simulink model "expertSystem"  (R2020a)
settings: Solver=ode45  StartTime=0.0  StopTime=0.25  FixedStep=1e-2  MaxStep=1e-2  RelTol=1e-3  EnableMultiTasking=on
StartFcn:
  | close all
StopFcn:
  | myStop()
libraries: simulink x15
settings Model: SimulationMode=accelerator  Creator=marcelo  LastModifiedBy=debora
settings SolverCC: ZeroCrossAlgorithm=Non-adaptive  AlgebraicLoopSolver=LineSearch
settings DataIOCC: SaveFormat=Array  SignalLoggingSaveFormat=ModelDataLogs  SaveOutput=off  ReturnWorkspaceOutputs=off
settings OptimizationCC: ExpressionDepthLimit=2147483647  InitFltsAndDblsToZero=on  LifeSpan=inf
settings DebuggingCC: SaveWithParameterizedLinksMsg=none  UnderspecifiedInitializationDetection=Classic  MergeDetectMultiDrivingBlocksExec=none  SignalResolutionControl=TryResolveAllWithWarning  SolverPrmCheckMsg=warning  MultiTaskDSMMsg=warning  MultiTaskCondExecSysMsg=none  FcnCallInpInsideContextMsg=warning  StateNameClashWarn=warning  SFUnexpectedBacktrackingDiag=warning  SFNoUnconditionalDefaultTransitionDiag=warning  SFExecutionAtInitializationDiag=none  ArithmeticOperatorsInVariantConditions=warning
settings HardwareCC: ProdBitPerPointer=32  ProdBitPerSizeT=32  ProdBitPerPtrDiffT=32  ProdLargestAtomicFloat=None  ProdIntDivRoundTo=Undefined  ProdEndianess=Unspecified  ProdWordSize=32  ProdHWDeviceType=32-bit Generic
settings ModelReferenceCC: PropagateSignalLabelsOutOfModel=off
settings CodeAppCC: StateflowObjectComments=on
settings GRTTargetCC: TargetFcnLib=ansi_tfl_tmw.mat  TargetLangStandard=C89/C90 (ANSI)  CombineOutputUpdateFcns=off  GRTInterface=on
settings ConfigComp: CovMetricSettings=dw  CovHtmlReporting=on  CovSaveCumulativeToWorkspaceVar=on  CovSaveSingleToWorkspaceVar=on

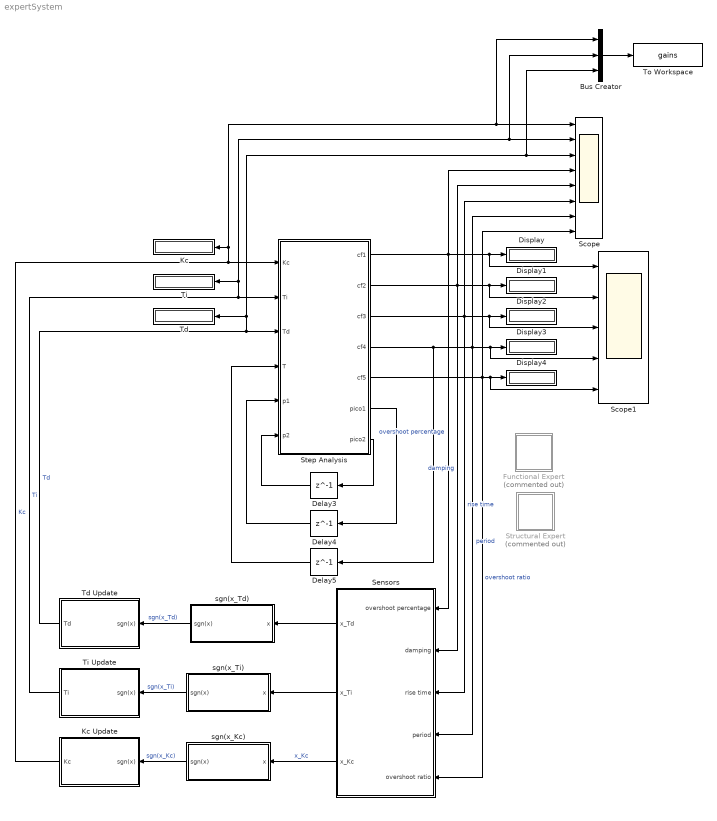
== system expertSystem ==
  Bus Creator : BusCreator  Inputs=3
  Delay3 : Delay  DelayLength=1
  Delay4 : Delay  DelayLength=1
  Delay5 : Delay  DelayLength=1
  Display{,1..4} (5 alike) : Display
  Functional Expert : Subsystem  Commented=on
  Kc : Display
  Kc Update : Subsystem
  Scope : Scope  NumInputPorts=8
  Scope1 : Scope  NumInputPorts=5
  Sensors : Subsystem
  Step Analysis : MATLAB Function  TreatAsAtomicUnit=on
  Structural Expert : Subsystem  Commented=on
  Td : Display
  Td Update : Subsystem
  Ti : Display
  Ti Update : Subsystem
  To Workspace : ToWorkspace  VariableName=gains  SampleTime=-1
      settings: Save2DSignal=2-D array (concatenate along first dimension)
  sgn(x_Kc) : Subsystem
  sgn(x_Td) : Subsystem
  sgn(x_Ti) : Subsystem
  wires:
  Step Analysis/1(cf1) -> Scope/4, Scope1/1, Display/1, Sensors/1(overshoot percentage)  "overshoot percentage"
  Step Analysis/2(cf2) -> Sensors/2(damping), Scope/5, Scope1/2, Display1/1  "damping"
  Step Analysis/3(cf3) -> Scope1/3, Display2/1, Sensors/3(rise time), Scope/6  "rise time"
  Step Analysis/4(cf4) -> Delay5/1, Sensors/4(period), Scope/7, Scope1/4, Display3/1  "period"
  Step Analysis/5(cf5) -> Sensors/5(overshoot ratio), Scope/8, Scope1/5, Display4/1  "overshoot ratio"
  Step Analysis/7(pico2) -> Delay3/1
  Step Analysis/6(pico1) -> Delay4/1
  Delay3/1 -> Step Analysis/6(p2)
  Delay4/1 -> Step Analysis/5(p1)
  Delay5/1 -> Step Analysis/4(T)
  Td Update/1(Td) -> Step Analysis/3(Td), Bus Creator/3, Scope/3, Td/1  "Td"
  Sensors/3(x_Kc) -> sgn(x_Kc)/1(x)  "x_Kc"
  sgn(x_Kc)/1(sgn(x)) -> Kc Update/1(sgn(x))  "sgn(x_Kc)"
  Kc Update/1(Kc) -> Bus Creator/1, Scope/1, Kc/1, Step Analysis/1(Kc)  "Kc"
  Sensors/2(x_Ti) -> sgn(x_Ti)/1(x)
  Sensors/1(x_Td) -> sgn(x_Td)/1(x)
  sgn(x_Td)/1(sgn(x)) -> Td Update/1(sgn(x))  "sgn(x_Td)"
  sgn(x_Ti)/1(sgn(x)) -> Ti Update/1(sgn(x))  "sgn(x_Ti)"
  Ti Update/1(Ti) -> Step Analysis/2(Ti), Bus Creator/2, Scope/2, Ti/1  "Ti"
  Bus Creator/1 -> To Workspace/1

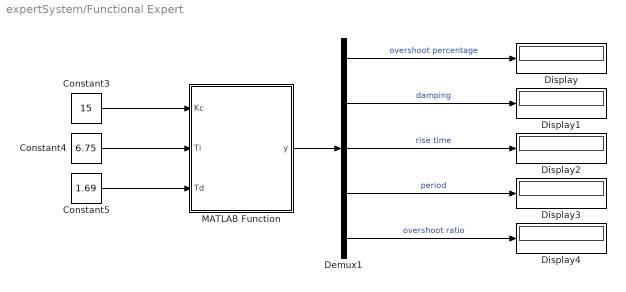
== system expertSystem/Functional Expert ==
  Constant3 : Constant  Value=15
  Constant4 : Constant  Value=6.75
  Constant5 : Constant  Value=1.69
  Demux1 : Demux  Outputs=5
  Display{,1..4} (5 alike) : Display
  MATLAB Function : MATLAB Function  TreatAsAtomicUnit=on
  wires:
  MATLAB Function/1(y) -> Demux1/1
  Demux1/4 -> Display3/1  "period"
  Demux1/3 -> Display2/1  "rise time"
  Demux1/1 -> Display/1  "overshoot percentage"
  Demux1/5 -> Display4/1  "overshoot ratio"
  Constant5/1 -> MATLAB Function/3(Td)
  Demux1/2 -> Display1/1  "damping"
  Constant3/1 -> MATLAB Function/1(Kc)
  Constant4/1 -> MATLAB Function/2(Ti)

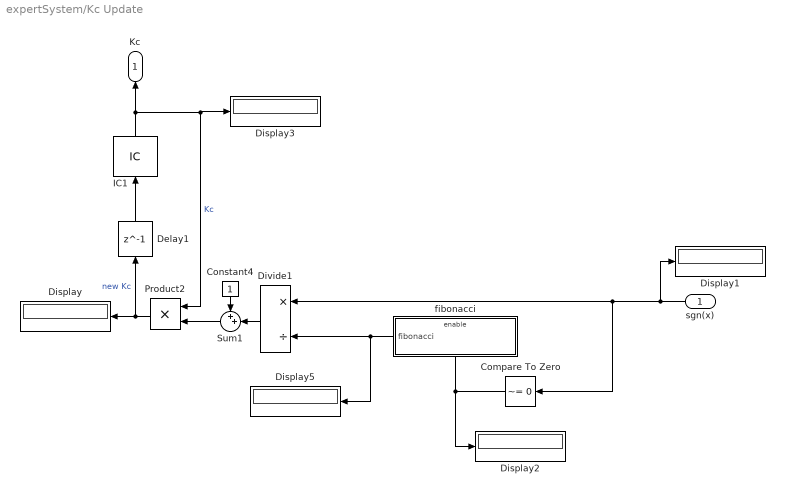
== system expertSystem/Kc Update ==
  sgn(x) : Inport
  Compare To Zero : simulink/Logic and Bit Operations/Compare To Zero  relop=~=  OutDataTypeStr=boolean
  Constant4 : Constant
  Delay1 : Delay  DelayLength=1
  Display{,1..3,5} (5 alike) : Display
  Divide1 : Product  Inputs=*/
  IC1 : InitialCondition  Value=15
  Product2 : Product
  Sum1 : Sum  Inputs=++|
  fibonacci : Subsystem
  Kc : Outport
  wires:
  IC1/1 -> Product2/1, Display3/1, Kc/1  "Kc"
  Delay1/1 -> IC1/1
  Compare To Zero/1 -> fibonacci/Enable, Display2/1
  fibonacci/1(fibonacci) -> Display5/1, Divide1/2
  Constant4/1 -> Sum1/1
  Sum1/1 -> Product2/2
  Divide1/1 -> Sum1/2
  Product2/1 -> Display/1, Delay1/1  "new Kc"
  sgn(x)/1 -> Display1/1, Divide1/1, Compare To Zero/1

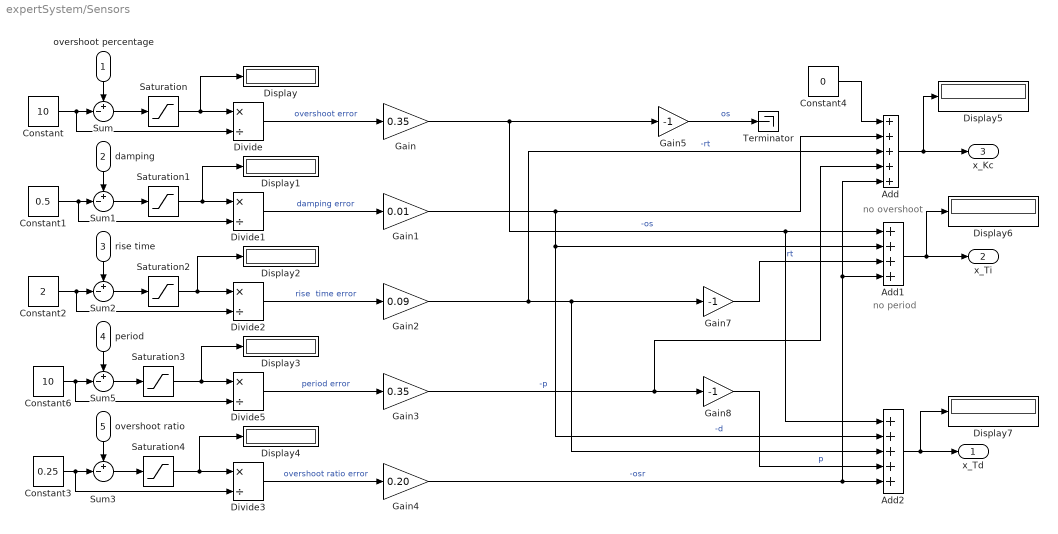
== system expertSystem/Sensors ==
  note: no overshoot
  note: no period
  overshoot percentage : Inport
  damping : Inport  Port=2
  rise time : Inport  Port=3
  period : Inport  Port=4
  overshoot ratio : Inport  Port=5
  Add : Sum  Inputs=5
  Add1 : Sum  Inputs=4
  Add2 : Sum  Inputs=5
  Constant : Constant  Value=10
  Constant1 : Constant  Value=0.5
  Constant2 : Constant  Value=2
  Constant3 : Constant  Value=0.25
  Constant4 : Constant  Value=0
  Constant6 : Constant  Value=10
  Display{,1..7} (8 alike) : Display
  Divide{,1..3,5} (5 alike) : Product  Inputs=*/
  Gain : Gain  Gain=0.35
  Gain1 : Gain  Gain=0.01
  Gain2 : Gain  Gain=0.09
  Gain3 : Gain  Gain=0.35
  Gain4 : Gain  Gain=0.20
  Gain5 : Gain  Gain=-1
  Gain7 : Gain  Gain=-1
  Gain8 : Gain  Gain=-1
  Saturation : Saturate  UpperLimit=10  LowerLimit=-10
  Saturation1 : Saturate
  Saturation2 : Saturate  UpperLimit=2  LowerLimit=-2
  Saturation3 : Saturate  UpperLimit=10  LowerLimit=-10
  Saturation4 : Saturate  UpperLimit=0.25  LowerLimit=-0.25
  Sum{,1..3,5} (5 alike) : Sum  Inputs=+-|
  Terminator : Terminator
  x_Td : Outport
  x_Ti : Outport  Port=2
  x_Kc : Outport  Port=3
  wires:
  rise time/1 -> Sum2/1
  Constant/1 -> Divide/2, Sum/2
  overshoot percentage/1 -> Sum/1
  damping/1 -> Sum1/1
  Constant1/1 -> Divide1/2, Sum1/2
  Constant2/1 -> Divide2/2, Sum2/2
  Divide/1 -> Gain/1  "overshoot error"
  Sum/1 -> Saturation/1
  Divide1/1 -> Gain1/1  "damping error"
  Sum1/1 -> Saturation1/1
  Divide2/1 -> Gain2/1  "rise  time error"
  Sum2/1 -> Saturation2/1
  Saturation/1 -> Display/1, Divide/1
  Saturation1/1 -> Display1/1, Divide1/1
  Saturation2/1 -> Display2/1, Divide2/1
  Saturation3/1 -> Display3/1, Divide5/1
  Divide5/1 -> Gain3/1  "period error"
  Constant6/1 -> Divide5/2, Sum5/2
  Sum5/1 -> Saturation3/1
  period/1 -> Sum5/1
  Sum3/1 -> Saturation4/1
  Constant3/1 -> Divide3/2, Sum3/2
  overshoot ratio/1 -> Sum3/1
  Divide3/1 -> Gain4/1  "overshoot ratio error"
  Saturation4/1 -> Display4/1, Divide3/1
  Gain/1 -> Gain5/1, Add1/1, Add2/1  "-os"
  Gain1/1 -> Add/2, Add1/2, Add2/2  "-d"
  Gain2/1 -> Gain7/1, Add2/3, Add/3  "-rt"
  Gain3/1 -> Add/4, Gain8/1  "-p"
  Gain4/1 -> Add2/5, Add/5, Add1/4  "-osr"
  Gain5/1 -> Terminator/1  "os"
  Add/1 -> Display5/1, x_Kc/1
  Add1/1 -> Display6/1, x_Ti/1
  Add2/1 -> Display7/1, x_Td/1
  Gain7/1 -> Add1/3  "rt"
  Gain8/1 -> Add2/4  "p"
  Constant4/1 -> Add/1

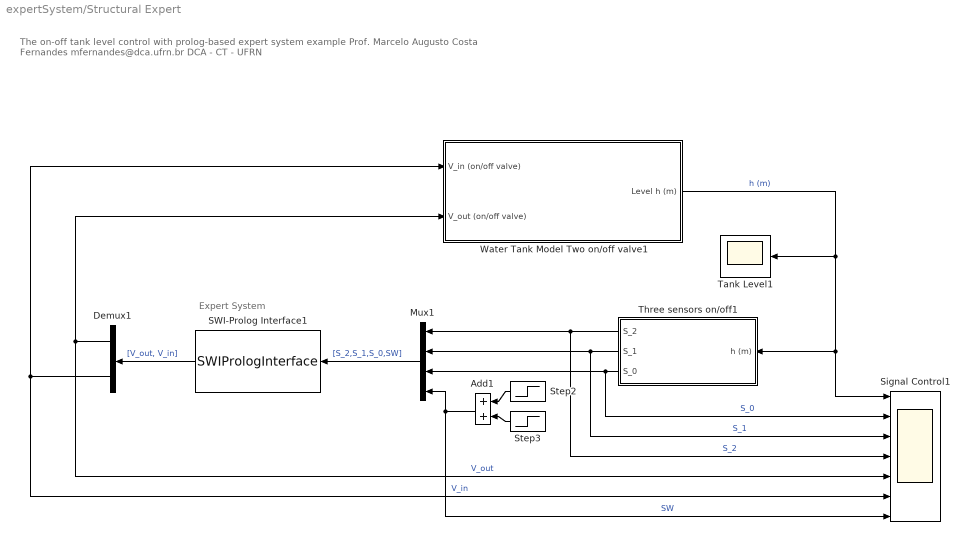
== system expertSystem/Structural Expert ==
  note: Expert System
  note: The on-off tank level control with prolog-based expert system example
      | Prof. Marcelo Augusto Costa Fernandes
      | mfernandes@dca.ufrn.br
      | DCA - CT - UFRN
  Add1 : Sum
  Demux1 : Demux  Outputs=2
  Mux1 : Mux
  SWI-Prolog Interface1 : S-Function  FunctionName=SWIPrologInterface  Parameters=jplPath, plFile, nIn, plQuery, nOut,0  SFunctionDeploymentMode=off  EnableBusSupport=off  mask(SWI-Prolog (www.swi-prolog.org) Interface){jplPath=C:\Arquivos de programas\swipl\lib\jpl.jar, plFile=example1Prolog.pl, nIn=4, nOut=2, plQuery=control(y(2),y(1),u(3),u(2),u(1),u(4))}
      mask prompts: jplPath "Path of the JPL jar-file:"; plFile "Prolog file:"; nIn "Number of the inputs:"; nOut "Number of the outputs:"; plQuery "Prolog query:"
      mask help:
      | SWI-Prolog (www.swi-prolog.org) Interface block.
      |
      | Execute Prolog code (PL file) in the Simulink environment.
      |
      | Use ''u'' as the input variable name and ''y'' as the output variable name.
      |
      | In the case of queries with multiple solutions, this block will only return the first solution found.
      |
      | Prof. Marcelo Augusto Costa Fernandes
      | mfernandes@dca.ufrn.br
      | DCA - CT - UFRN
      mask Help:
      | SWI-Prolog (www.swi-prolog.org) Interface block.
      | 
      | Execute Prolog code (PL file) in the Simulink environment.
      | 
      | Use ''u'' as the input variable name and ''y'' as the output variable name.
      | 
      | In the case of queries with multiple solutions, this block will only return the first solution found.
      | 
      | Prof. Marcelo Augusto Costa Fernandes
      | mfernandes@dca.ufrn.br
      | DCA - CT - UFRN
      mask Display: disp('SWI-Prolog\nInterface')
  Signal Control1 : Scope  NumInputPorts=7
  Step2 : Step  SampleTime=0
  Step3 : Step  Time=8  After=-1  SampleTime=0
  Tank Level1 : Scope
  Three sensors on/off1 : Subsystem
      mask Display: disp('Three sensors\non/off')
  Water Tank Model Two on/off valve1 : Subsystem  mask(Water Tank Model){q1=1, h=2, area=1, outletArea=.1}
      mask prompts: q1 "Input flow - q_1 (m^3/s)"; h "Tank height - H (m):"; area "Area - A (m^2):"; outletArea "outlet area (m^2):"
      mask help:
      | Water tank model with two on/off valve: V_in and V_out.
      | V_in is the input valve and V_out is the output valve.
      |
      | Prof. Marcelo Augusto C. Fernandes
      | mfernandes@dca.ufrn.br
      | DCA - CT - UFRN
      mask Display: disp('Water Tank Model\nTwo on/off valve')
  wires:
  Demux1/1 -> Water Tank Model Two on/off valve1/2(V_out (on/off valve)), Signal Control1/5  "V_out"
  Three sensors on/off1/1(S_2) -> Signal Control1/4, Mux1/1  "S_2"
  Add1/1 -> Mux1/4, Signal Control1/7  "SW"
  Water Tank Model Two on/off valve1/1(Level h (m)) -> Signal Control1/1, Three sensors on/off1/1(h (m)), Tank Level1/1  "h (m)"
  Step2/1 -> Add1/1
  SWI-Prolog Interface1/1 -> Demux1/1  "[V_out, V_in]"
  Mux1/1 -> SWI-Prolog Interface1/1  "[S_2,S_1,S_0,SW]"
  Step3/1 -> Add1/2
  Three sensors on/off1/2(S_1) -> Signal Control1/3, Mux1/2  "S_1"
  Demux1/2 -> Water Tank Model Two on/off valve1/1(V_in (on/off valve)), Signal Control1/6  "V_in"
  Three sensors on/off1/3(S_0) -> Signal Control1/2, Mux1/3  "S_0"

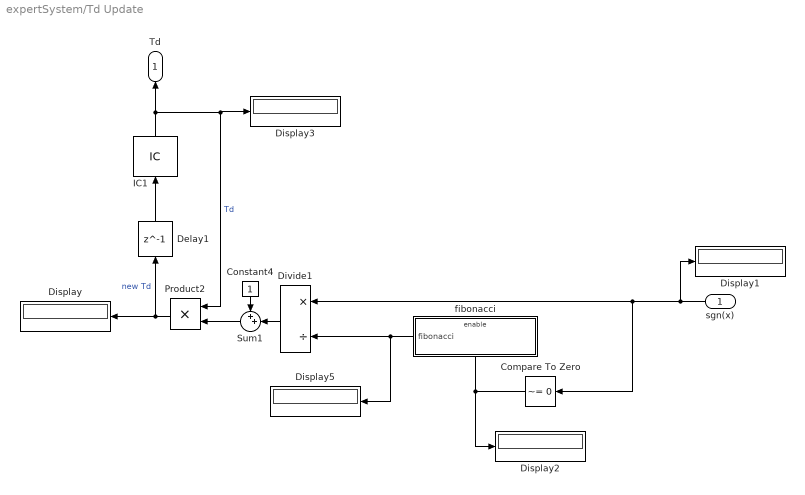
== system expertSystem/Td Update ==
  sgn(x) : Inport
  Compare To Zero : simulink/Logic and Bit Operations/Compare To Zero  relop=~=  OutDataTypeStr=boolean
  Constant4 : Constant
  Delay1 : Delay  DelayLength=1
  Display{,1..3,5} (5 alike) : Display
  Divide1 : Product  Inputs=*/
  IC1 : InitialCondition  Value=1.69
  Product2 : Product
  Sum1 : Sum  Inputs=++|
  fibonacci : Subsystem
  Td : Outport
  wires:
  IC1/1 -> Product2/1, Display3/1, Td/1  "Td"
  Delay1/1 -> IC1/1
  Compare To Zero/1 -> fibonacci/Enable, Display2/1
  fibonacci/1(fibonacci) -> Display5/1, Divide1/2
  Constant4/1 -> Sum1/1
  Sum1/1 -> Product2/2
  Divide1/1 -> Sum1/2
  Product2/1 -> Display/1, Delay1/1  "new Td"
  sgn(x)/1 -> Display1/1, Divide1/1, Compare To Zero/1

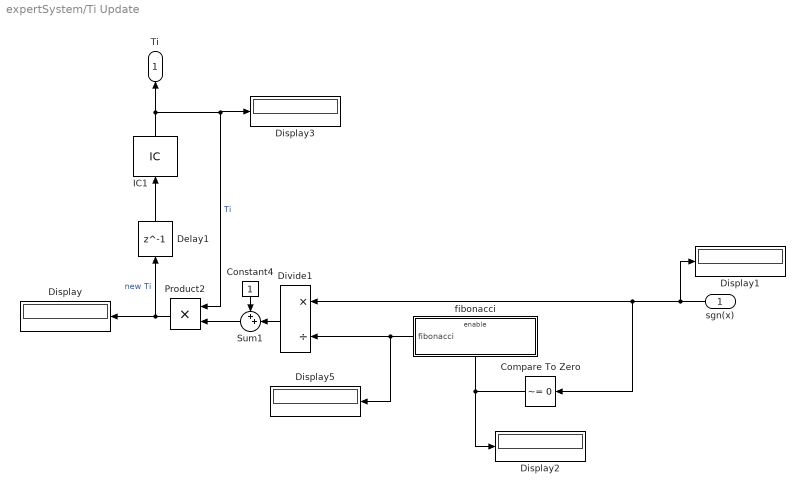
== system expertSystem/Ti Update ==
  sgn(x) : Inport
  Compare To Zero : simulink/Logic and Bit Operations/Compare To Zero  relop=~=  OutDataTypeStr=boolean
  Constant4 : Constant
  Delay1 : Delay  DelayLength=1
  Display{,1..3,5} (5 alike) : Display
  Divide1 : Product  Inputs=*/
  IC1 : InitialCondition  Value=6.75
  Product2 : Product
  Sum1 : Sum  Inputs=++|
  fibonacci : Subsystem
  Ti : Outport
  wires:
  IC1/1 -> Product2/1, Display3/1, Ti/1  "Ti"
  Delay1/1 -> IC1/1
  Compare To Zero/1 -> fibonacci/Enable, Display2/1
  fibonacci/1(fibonacci) -> Display5/1, Divide1/2
  Constant4/1 -> Sum1/1
  Sum1/1 -> Product2/2
  Divide1/1 -> Sum1/2
  Product2/1 -> Display/1, Delay1/1  "new Ti"
  sgn(x)/1 -> Display1/1, Divide1/1, Compare To Zero/1

== system expertSystem/sgn(x_Kc) ==
  x : Inport
  Add : Sum  Inputs=2
  Compare To Constant : simulink/Logic and Bit Operations/Compare To Constant  relop=<  const=0.01  OutDataTypeStr=boolean
  Compare To Constant1 : simulink/Logic and Bit Operations/Compare To Constant  relop=>  const=0.01  OutDataTypeStr=boolean
  Data Type Conversion : DataTypeConversion  OutDataTypeStr=double
  Data Type Conversion1 : DataTypeConversion  OutDataTypeStr=double
  Gain : Gain  Gain=-1
  sgn(x) : Outport
  wires:
  Compare To Constant/1 -> Data Type Conversion1/1
  Compare To Constant1/1 -> Data Type Conversion/1
  Gain/1 -> Add/1
  x/1 -> Compare To Constant/1, Compare To Constant1/1
  Add/1 -> sgn(x)/1
  Data Type Conversion1/1 -> Gain/1
  Data Type Conversion/1 -> Add/2

== system expertSystem/sgn(x_Td) ==
  x : Inport
  Add : Sum  Inputs=2
  Compare To Constant : simulink/Logic and Bit Operations/Compare To Constant  relop=<  const=0.01  OutDataTypeStr=boolean
  Compare To Constant1 : simulink/Logic and Bit Operations/Compare To Constant  relop=>  const=0.01  OutDataTypeStr=boolean
  Data Type Conversion : DataTypeConversion  OutDataTypeStr=double
  Data Type Conversion1 : DataTypeConversion  OutDataTypeStr=double
  Gain : Gain  Gain=-1
  sgn(x) : Outport
  wires:
  Compare To Constant/1 -> Data Type Conversion1/1
  Compare To Constant1/1 -> Data Type Conversion/1
  Gain/1 -> Add/1
  x/1 -> Compare To Constant1/1, Compare To Constant/1
  Add/1 -> sgn(x)/1
  Data Type Conversion1/1 -> Gain/1
  Data Type Conversion/1 -> Add/2

== system expertSystem/sgn(x_Ti) ==
  x : Inport
  Add : Sum  Inputs=2
  Compare To Constant : simulink/Logic and Bit Operations/Compare To Constant  relop=<  const=0.01  OutDataTypeStr=boolean
  Compare To Constant1 : simulink/Logic and Bit Operations/Compare To Constant  relop=>  const=0.01  OutDataTypeStr=boolean
  Data Type Conversion : DataTypeConversion  OutDataTypeStr=double
  Data Type Conversion1 : DataTypeConversion  OutDataTypeStr=double
  Gain : Gain  Gain=-1
  sgn(x) : Outport
  wires:
  Compare To Constant/1 -> Data Type Conversion1/1
  Compare To Constant1/1 -> Data Type Conversion/1
  Gain/1 -> Add/1
  x/1 -> Compare To Constant1/1, Compare To Constant/1
  Add/1 -> sgn(x)/1
  Data Type Conversion1/1 -> Gain/1
  Data Type Conversion/1 -> Add/2

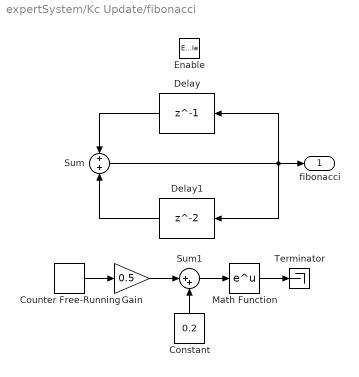
== system expertSystem/Kc Update/fibonacci ==
  Enable : EnablePort  PropagateVarSize=During execution
  Constant : Constant  Value=0.2
  Counter Free-Running : simulink/Sources/Counter Free-Running  NumBits=16  tsamp=-1
  Delay : Delay  DelayLength=1  InitialCondition=0  InputProcessing=Columns as channels (frame based)
  Delay1 : Delay  InitialCondition=1.2  InputProcessing=Columns as channels (frame based)
  Gain : Gain  Gain=0.5
  Math Function : Math  SaturateOnIntegerOverflow=on
  Sum : Sum  Inputs=+|+
  Sum1 : Sum  Inputs=|++
  Terminator : Terminator
  fibonacci : Outport  InitialOutput=1
  wires:
  Delay1/1 -> Sum/2
  Delay/1 -> Sum/1
  Sum1/1 -> Math Function/1
  Counter Free-Running/1 -> Gain/1
  Gain/1 -> Sum1/1
  Constant/1 -> Sum1/2
  Sum/1 -> fibonacci/1, Delay/1, Delay1/1
  Math Function/1 -> Terminator/1

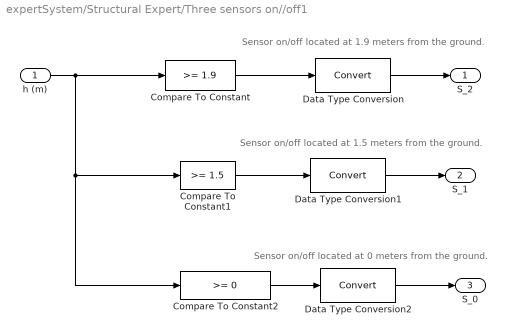
== system expertSystem/Structural Expert/Three sensors on//off1 ==
  note: Sensor on/off located at 0 meters from the ground.
  note: Sensor on/off located at 1.5 meters from the ground.
  note: Sensor on/off located at 1.9 meters from the ground.
  h (m) : Inport
  Compare To Constant : simulink/Logic and Bit Operations/Compare To Constant  relop=>=  const=1.9  OutDataTypeStr=boolean  ZeroCross=off
  Compare To Constant1 : simulink/Logic and Bit Operations/Compare To Constant  relop=>=  const=1.5  OutDataTypeStr=boolean  ZeroCross=off
  Compare To Constant2 : simulink/Logic and Bit Operations/Compare To Constant  relop=>=  const=0  OutDataTypeStr=boolean  ZeroCross=off
  Data Type Conversion : DataTypeConversion
  Data Type Conversion1 : DataTypeConversion
  Data Type Conversion2 : DataTypeConversion
  S_2 : Outport
  S_1 : Outport  Port=2
  S_0 : Outport  Port=3
  wires:
  h (m)/1 -> Compare To Constant/1, Compare To Constant1/1, Compare To Constant2/1
  Compare To Constant/1 -> Data Type Conversion/1
  Compare To Constant2/1 -> Data Type Conversion2/1
  Compare To Constant1/1 -> Data Type Conversion1/1
  Data Type Conversion/1 -> S_2/1
  Data Type Conversion1/1 -> S_1/1
  Data Type Conversion2/1 -> S_0/1

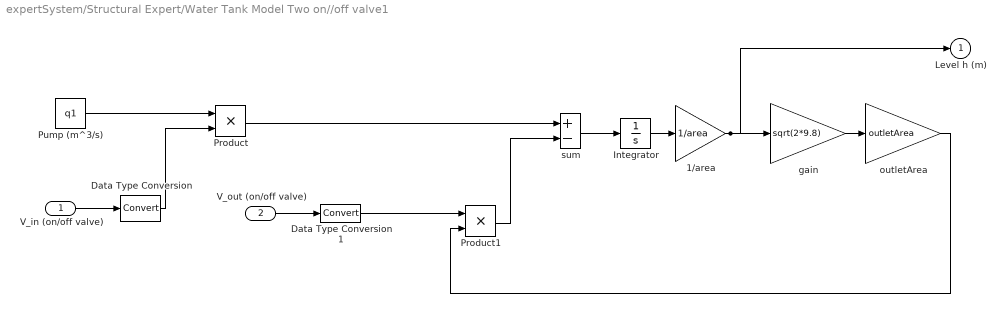
== system expertSystem/Structural Expert/Water Tank Model Two on//off valve1 ==
  V_in (on/off valve) : Inport
  V_out (on/off valve) : Inport  Port=2
  1/area : Gain  Gain=1/area  SaturateOnIntegerOverflow=on  OutDataTypeStr=Inherit: Same as input  ParamDataTypeStr=Inherit: Same as input
  Data Type Conversion : DataTypeConversion
  Data Type Conversion1 : DataTypeConversion
  Integrator : Integrator
  Product : Product  RndMeth=Zero  OutDataTypeStr=Inherit: Same as first input
  Product1 : Product  RndMeth=Zero  OutDataTypeStr=Inherit: Same as first input
  Pump (m^3/s) : Constant  Value=q1
  gain : Gain  Gain=sqrt(2*9.8)  SaturateOnIntegerOverflow=on  OutDataTypeStr=Inherit: Same as input  ParamDataTypeStr=Inherit: Same as input
  outletArea : Gain  Gain=outletArea  SaturateOnIntegerOverflow=on  OutDataTypeStr=Inherit: Same as input  ParamDataTypeStr=Inherit: Same as input
  sum : Sum  Inputs=+-  InputSameDT=on  SaturateOnIntegerOverflow=on  OutDataTypeStr=Inherit: Same as first input
  Level h (m) : Outport  InitialOutput=0
  wires:
  outletArea/1 -> Product1/2
  gain/1 -> outletArea/1
  1/area/1 -> Level h (m)/1, gain/1
  Integrator/1 -> 1/area/1
  Product/1 -> sum/1
  sum/1 -> Integrator/1
  Pump (m^3/s)/1 -> Product/1
  V_in (on/off valve)/1 -> Data Type Conversion/1
  Product1/1 -> sum/2
  Data Type Conversion1/1 -> Product1/1
  V_out (on/off valve)/1 -> Data Type Conversion1/1
  Data Type Conversion/1 -> Product/2

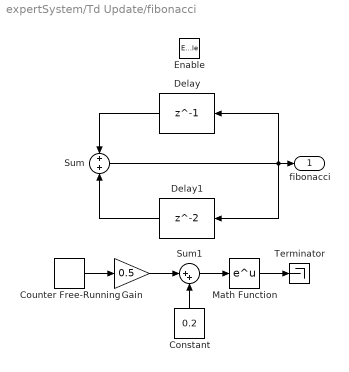
== system expertSystem/Td Update/fibonacci ==
  Enable : EnablePort  PropagateVarSize=During execution
  Constant : Constant  Value=0.2
  Counter Free-Running : simulink/Sources/Counter Free-Running  NumBits=16  tsamp=-1
  Delay : Delay  DelayLength=1  InitialCondition=0  InputProcessing=Columns as channels (frame based)
  Delay1 : Delay  InitialCondition=1.2  InputProcessing=Columns as channels (frame based)
  Gain : Gain  Gain=0.5
  Math Function : Math  SaturateOnIntegerOverflow=on
  Sum : Sum  Inputs=+|+
  Sum1 : Sum  Inputs=|++
  Terminator : Terminator
  fibonacci : Outport  InitialOutput=1
  wires:
  Delay1/1 -> Sum/2
  Delay/1 -> Sum/1
  Sum/1 -> fibonacci/1, Delay/1, Delay1/1
  Sum1/1 -> Math Function/1
  Constant/1 -> Sum1/2
  Counter Free-Running/1 -> Gain/1
  Gain/1 -> Sum1/1
  Math Function/1 -> Terminator/1

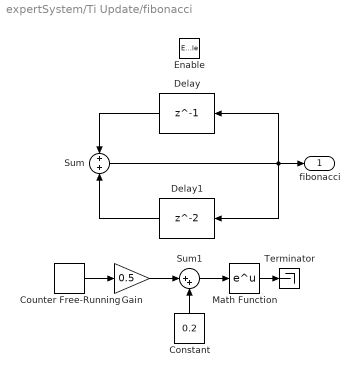
== system expertSystem/Ti Update/fibonacci ==
  Enable : EnablePort  PropagateVarSize=During execution
  Constant : Constant  Value=0.2
  Counter Free-Running : simulink/Sources/Counter Free-Running  NumBits=16  tsamp=-1
  Delay : Delay  DelayLength=1  InitialCondition=0  InputProcessing=Columns as channels (frame based)
  Delay1 : Delay  InitialCondition=1.2  InputProcessing=Columns as channels (frame based)
  Gain : Gain  Gain=0.5
  Math Function : Math  SaturateOnIntegerOverflow=on
  Sum : Sum  Inputs=+|+
  Sum1 : Sum  Inputs=|++
  Terminator : Terminator
  fibonacci : Outport  InitialOutput=1
  wires:
  Delay1/1 -> Sum/2
  Delay/1 -> Sum/1
  Sum/1 -> fibonacci/1, Delay/1, Delay1/1
  Sum1/1 -> Math Function/1
  Constant/1 -> Sum1/2
  Counter Free-Running/1 -> Gain/1
  Gain/1 -> Sum1/1
  Math Function/1 -> Terminator/1

== matlab function expertSystem/Functional Expert/MATLAB Function ==
  data: Kc input; y output; Ti input; Td input
function y = fcn(Kc,Ti,Td)
    y = ones(5,1);
    coder.extrinsic('myExpert');
    [cf1,cf2,cf3,cf4,cf5] = myExpert(Kc,Ti,Td);
    y = [cf1,cf2,cf3,cf4,cf5];

== matlab function expertSystem/Step Analysis ==
  data: Kc input; cf1 output; Ti input; Td input; T input; cf2 output; cf3 output; cf4 output; cf5 output; pico1 output; pico2 output; p1 input; p2 input
function [cf1,cf2,cf3,cf4,cf5,pico1,pico2] = fcn(Kc,Ti,Td,T,p1,p2)
    cf1 = 0;
    cf2 = 0;
    cf3 = 0;
    cf4 = 0;
    cf5 = 0;
    pico1 = 0;
    pico2 = 0;
    coder.extrinsic('myExpert');
    [cf1,cf2,cf3,cf4,cf5,pico1,pico2] = myExpert(Kc,Ti,Td,p1,p2,T);
